simulink model "Tut5_SimulinkIntro"  (R2021a)
settings: Solver=VariableStepAuto  StartTime=0.0  StopTime=10.0  RelTol=1e-3
settings Model: Creator=cheta  LastModifiedBy=cheta

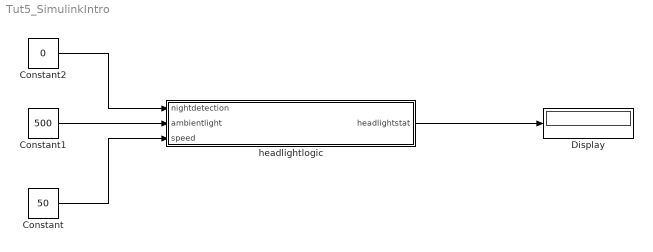
== system Tut5_SimulinkIntro ==
  Constant : Constant  Value=50
  Constant1 : Constant  Value=500
  Constant2 : Constant  Value=0
  Display : Display
  headlightlogic : Subsystem
  wires:
  headlightlogic/1(headlightstat) -> Display/1
  Constant2/1 -> headlightlogic/1(nightdetection)
  Constant1/1 -> headlightlogic/2(ambientlight)
  Constant/1 -> headlightlogic/3(speed)

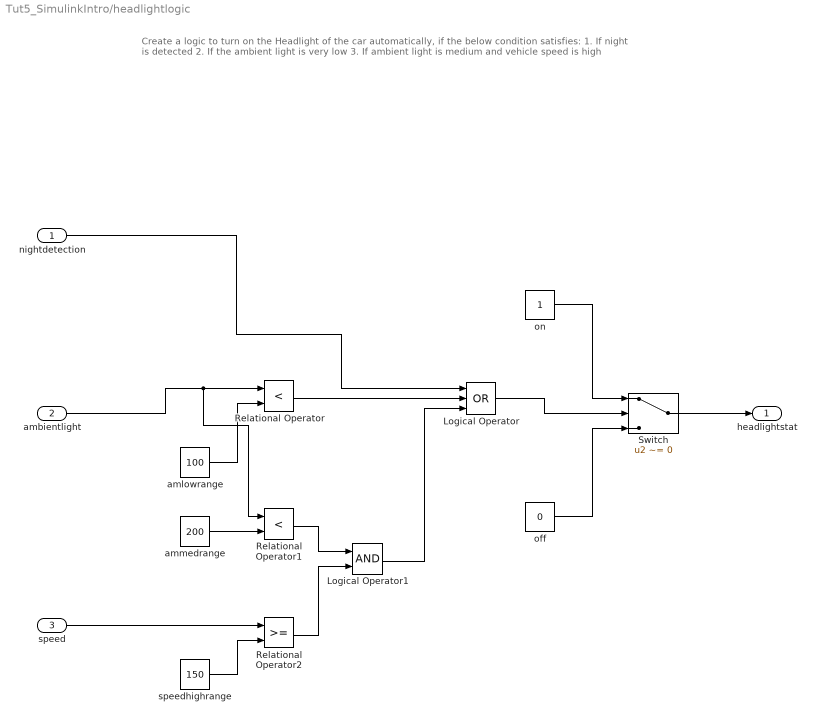
== system Tut5_SimulinkIntro/headlightlogic ==
  note: Create a logic to turn on the Headlight of the car automatically, if the below condition satisfies:
      | 1.	If night is detected
      | 2.	If the ambient light is very low
      | 3.	If ambient light is medium and vehicle speed is high
  nightdetection : Inport
  ambientlight : Inport  Port=2
  speed : Inport  Port=3
  Logical Operator : Logic  Operator=OR  Inputs=3  AllPortsSameDT=off  OutDataTypeStr=boolean
  Logical Operator1 : Logic  AllPortsSameDT=off  OutDataTypeStr=boolean
  Relational Operator : RelationalOperator  Operator=<  OutDataTypeStr=boolean  RndMeth=Simplest
  Relational Operator1 : RelationalOperator  Operator=<  OutDataTypeStr=boolean  RndMeth=Simplest
  Relational Operator2 : RelationalOperator  OutDataTypeStr=boolean  RndMeth=Simplest
  Switch : Switch  Criteria=u2 ~= 0
  amlowrange : Constant  Value=100
  ammedrange : Constant  Value=200
  off : Constant  Value=0
  on : Constant
  speedhighrange : Constant  Value=150
  headlightstat : Outport
  wires:
  Switch/1 -> headlightstat/1
  on/1 -> Switch/1
  off/1 -> Switch/3
  ambientlight/1 -> Relational Operator1/1, Relational Operator/1
  amlowrange/1 -> Relational Operator/2
  nightdetection/1 -> Logical Operator/1
  Relational Operator/1 -> Logical Operator/2
  Logical Operator/1 -> Switch/2
  ammedrange/1 -> Relational Operator1/2
  speed/1 -> Relational Operator2/1
  speedhighrange/1 -> Relational Operator2/2
  Relational Operator1/1 -> Logical Operator1/1
  Relational Operator2/1 -> Logical Operator1/2
  Logical Operator1/1 -> Logical Operator/3
